simulink model "Tracking_04"  (R2022b)
settings: Solver=ode4  StartTime=0.0  StopTime=50  FixedStep=1e-3  MaxStep=1e-3  RelTol=1e-3
undefined symbols (not defined in the file or in its folder): SF_a, SF_xi2, TT_theta1_init, TT_theta2_init, TT_theta3_init, TT_x_init, TT_y_init, v_sat, w_sat
libraries: simulink x18, dspsigops x3
settings Model: Creator=david  LastModifiedBy=david

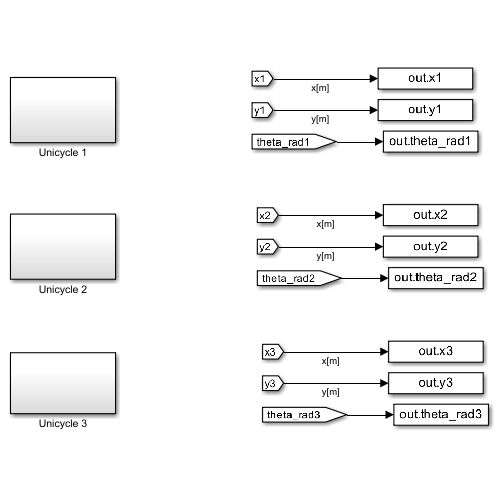
[thumbnail: Simulink's stored preview of the top-level diagram]
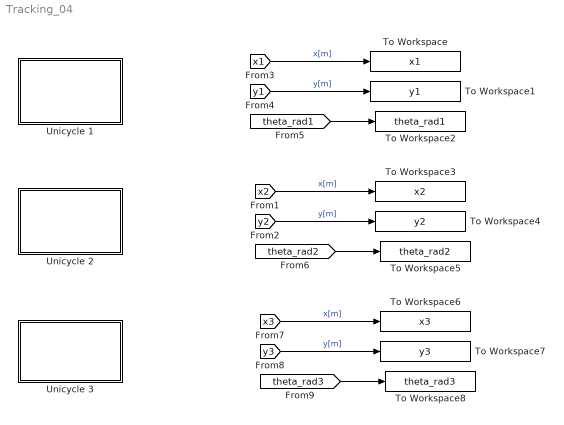
== system Tracking_04 ==
  To Workspace : ToWorkspace  VariableName=x1  SaveFormat=Structure With Time  SampleTime=-1
  To Workspace1 : ToWorkspace  VariableName=y1  SaveFormat=Structure With Time  SampleTime=-1
  To Workspace2 : ToWorkspace  VariableName=theta_rad1  SaveFormat=Structure With Time  SampleTime=-1
  To Workspace3 : ToWorkspace  VariableName=x2  SaveFormat=Structure With Time  SampleTime=-1
  To Workspace4 : ToWorkspace  VariableName=y2  SaveFormat=Structure With Time  SampleTime=-1
  To Workspace5 : ToWorkspace  VariableName=theta_rad2  SaveFormat=Structure With Time  SampleTime=-1
  To Workspace6 : ToWorkspace  VariableName=x3  SaveFormat=Structure With Time  SampleTime=-1
  To Workspace7 : ToWorkspace  VariableName=y3  SaveFormat=Structure With Time  SampleTime=-1
  To Workspace8 : ToWorkspace  VariableName=theta_rad3  SaveFormat=Structure With Time  SampleTime=-1
  Unicycle 1 : Subsystem
  Unicycle 2 : Subsystem
  Unicycle 3 : Subsystem
  wires:
  [x1] -> To Workspace/1  "x[m]"
  [y1] -> To Workspace1/1  "y[m]"
  [theta_rad1] -> To Workspace2/1
  [x2] -> To Workspace3/1  "x[m]"
  [y2] -> To Workspace4/1  "y[m]"
  [theta_rad2] -> To Workspace5/1
  [theta_rad3] -> To Workspace8/1
  [y3] -> To Workspace7/1  "y[m]"
  [x3] -> To Workspace6/1  "x[m]"

== system Tracking_04/Unicycle 1 ==
  State Feedback Approximate Trajectory Controller : Subsystem
  To Workspace : ToWorkspace  VariableName=v1  SaveFormat=Structure With Time  SampleTime=-1
  To Workspace1 : ToWorkspace  VariableName=w1  SaveFormat=Structure With Time  SampleTime=-1
  "Trajectory Generator 1 " : Subsystem
  Unicycle Kinematics : Subsystem
  tag scope: theta_rad1=global, x1=global, y1=global
  wires:
  Unicycle Kinematics/3(theta[rad]) -> [theta_rad1]  "theta[rad]"
  Unicycle Kinematics/2(y[m]) -> [y1]  "y[m]"
  Unicycle Kinematics/1(x[m]) -> [x1]  "x[m]"
  [theta_rad1] -> State Feedback Approximate Trajectory Controller/3(theta[rad])
  [x1] -> State Feedback Approximate Trajectory Controller/1(x[m])
  [y1] -> State Feedback Approximate Trajectory Controller/2(y[m])
  "Trajectory Generator 1 "/1(x_d) -> State Feedback Approximate Trajectory Controller/4(x_d)
  "Trajectory Generator 1 "/2(y_d) -> State Feedback Approximate Trajectory Controller/5(y_d)
  State Feedback Approximate Trajectory Controller/1(v) -> Unicycle Kinematics/1(v[m/s]), To Workspace/1
  State Feedback Approximate Trajectory Controller/2(w) -> Unicycle Kinematics/2(w[rad/s]), To Workspace1/1

== system Tracking_04/Unicycle 2 ==
  State Feedback Approcimate Trajectory Controller : Subsystem
  To Workspace : ToWorkspace  VariableName=v2  SaveFormat=Structure With Time  SampleTime=-1
  To Workspace1 : ToWorkspace  VariableName=w2  SaveFormat=Structure With Time  SampleTime=-1
  "Trajectory Generator 1 " : Subsystem
  Unicycle Kinematics : Subsystem
  tag scope: theta_rad2=global, x2=global, y2=global
  wires:
  Unicycle Kinematics/3(theta[rad]) -> [theta_rad2]  "theta[rad]"
  Unicycle Kinematics/2(y[m]) -> [y2]  "y[m]"
  Unicycle Kinematics/1(x[m]) -> [x2]  "x[m]"
  [theta_rad2] -> State Feedback Approcimate Trajectory Controller/3(theta[rad])
  [x2] -> State Feedback Approcimate Trajectory Controller/1(x[m])
  [y2] -> State Feedback Approcimate Trajectory Controller/2(y[m])
  "Trajectory Generator 1 "/1(x_d) -> State Feedback Approcimate Trajectory Controller/4(x_d)
  "Trajectory Generator 1 "/2(y_d) -> State Feedback Approcimate Trajectory Controller/5(y_d)
  State Feedback Approcimate Trajectory Controller/1(v) -> Unicycle Kinematics/1(v[m/s]), To Workspace/1
  State Feedback Approcimate Trajectory Controller/2(w) -> Unicycle Kinematics/2(w[rad/s]), To Workspace1/1

== system Tracking_04/Unicycle 3 ==
  State Feedback Approximate Trajectory Controller : Subsystem
  To Workspace : ToWorkspace  VariableName=v3  SaveFormat=Structure With Time  SampleTime=-1
  To Workspace1 : ToWorkspace  VariableName=w3  SaveFormat=Structure With Time  SampleTime=-1
  "Trajectory Generator 3 " : Subsystem
  Unicycle Kinematics : Subsystem
  tag scope: theta_rad3=global, x3=global, y3=global
  wires:
  Unicycle Kinematics/3(theta[rad]) -> [theta_rad3]  "theta[rad]"
  Unicycle Kinematics/2(y[m]) -> [y3]  "y[m]"
  Unicycle Kinematics/1(x[m]) -> [x3]  "x[m]"
  [theta_rad3] -> State Feedback Approximate Trajectory Controller/3(theta[rad])
  [x3] -> State Feedback Approximate Trajectory Controller/1(x[m])
  [y3] -> State Feedback Approximate Trajectory Controller/2(y[m])
  "Trajectory Generator 3 "/2(y_d) -> State Feedback Approximate Trajectory Controller/5(y_d)
  "Trajectory Generator 3 "/1(x_d) -> State Feedback Approximate Trajectory Controller/4(x_d)
  State Feedback Approximate Trajectory Controller/1(v) -> Unicycle Kinematics/1(v[m/s]), To Workspace/1
  State Feedback Approximate Trajectory Controller/2(w) -> Unicycle Kinematics/2(w[rad/s]), To Workspace1/1

== system Tracking_04/Unicycle 1/State Feedback Approximate Trajectory Controller ==
  x[m] : Inport
  y[m] : Inport  Port=2
  theta[rad] : Inport  Port=3
  x_d : Inport  Port=4
  y_d : Inport  Port=5
  Controller : Subsystem
  Differential Flatness : Subsystem
  Saturation : Saturate  UpperLimit=v_sat  LowerLimit=-v_sat
  Saturation1 : Saturate  UpperLimit=w_sat  LowerLimit=-w_sat
  v : Outport
  w : Outport  Port=2
  wires:
  Controller/2(w) -> Saturation1/1
  Controller/1(v) -> Saturation/1
  Differential Flatness/3(w_d) -> Controller/3(w_d)
  Differential Flatness/1(q_d) -> Controller/1(q_d)
  Differential Flatness/2(v_d) -> Controller/2(v_d)
  y_d/1 -> Differential Flatness/2(y_d)
  x_d/1 -> Differential Flatness/1(x_d)
  x[m]/1 -> Controller/4(x)
  y[m]/1 -> Controller/5(y)
  theta[rad]/1 -> Controller/6(theta)
  Saturation/1 -> v/1
  Saturation1/1 -> w/1

== system Tracking_04/Unicycle 1/Trajectory Generator 1  ==
  Repeating Sequence : simulink/Sources/Repeating Sequence  rep_seq_t=time  rep_seq_y=y_d1
  Repeating Sequence1 : simulink/Sources/Repeating Sequence  rep_seq_t=time  rep_seq_y=x_d1
  To Workspace2 : ToWorkspace  VariableName=y_d1  SaveFormat=Structure With Time  SampleTime=-1
  To Workspace3 : ToWorkspace  VariableName=x_d1  SaveFormat=Structure With Time  SampleTime=-1
  x_d : Outport
  y_d : Outport  Port=2
  wires:
  Repeating Sequence/1 -> y_d/1, To Workspace2/1
  Repeating Sequence1/1 -> x_d/1, To Workspace3/1

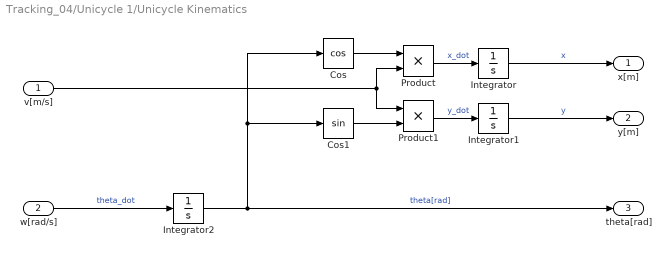
== system Tracking_04/Unicycle 1/Unicycle Kinematics ==
  v[m/s] : Inport
  w[rad/s] : Inport  Port=2
  Cos : Trigonometry  Operator=cos
  Cos1 : Trigonometry
  Integrator : Integrator  InitialCondition=TT_x_init
  Integrator1 : Integrator  InitialCondition=TT_y_init
  Integrator2 : Integrator  InitialCondition=TT_theta1_init
  Product : Product
  Product1 : Product
  x[m] : Outport
  y[m] : Outport  Port=2
  theta[rad] : Outport  Port=3
  wires:
  Integrator/1 -> x[m]/1  "x"
  Integrator1/1 -> y[m]/1  "y"
  w[rad/s]/1 -> Integrator2/1  "theta_dot"
  Integrator2/1 -> Cos/1, Cos1/1, theta[rad]/1  "theta[rad]"
  Product/1 -> Integrator/1  "x_dot"
  Cos1/1 -> Product1/2
  Cos/1 -> Product/1
  v[m/s]/1 -> Product1/1, Product/2
  Product1/1 -> Integrator1/1  "y_dot"

== system Tracking_04/Unicycle 2/State Feedback Approcimate Trajectory Controller ==
  x[m] : Inport
  y[m] : Inport  Port=2
  theta[rad] : Inport  Port=3
  x_d : Inport  Port=4
  y_d : Inport  Port=5
  Controller : Subsystem
  Differential Flatness : Subsystem
  Saturation : Saturate  UpperLimit=v_sat  LowerLimit=-v_sat
  Saturation1 : Saturate  UpperLimit=w_sat  LowerLimit=-w_sat
  v : Outport
  w : Outport  Port=2
  wires:
  Controller/2(w) -> Saturation1/1
  Controller/1(v) -> Saturation/1
  Differential Flatness/3(w_d) -> Controller/3(w_d)
  Differential Flatness/1(q_d) -> Controller/1(q_d)
  Differential Flatness/2(v_d) -> Controller/2(v_d)
  y_d/1 -> Differential Flatness/2(y_d)
  x_d/1 -> Differential Flatness/1(x_d)
  x[m]/1 -> Controller/4(x)
  y[m]/1 -> Controller/5(y)
  theta[rad]/1 -> Controller/6(theta)
  Saturation/1 -> v/1
  Saturation1/1 -> w/1

== system Tracking_04/Unicycle 2/Trajectory Generator 1  ==
  Repeating Sequence : simulink/Sources/Repeating Sequence  rep_seq_t=time  rep_seq_y=y_d2
  Repeating Sequence1 : simulink/Sources/Repeating Sequence  rep_seq_t=time  rep_seq_y=x_d2
  To Workspace2 : ToWorkspace  VariableName=y_d2  SaveFormat=Structure With Time  SampleTime=-1
  To Workspace3 : ToWorkspace  VariableName=x_d2  SaveFormat=Structure With Time  SampleTime=-1
  x_d : Outport
  y_d : Outport  Port=2
  wires:
  Repeating Sequence/1 -> y_d/1, To Workspace2/1
  Repeating Sequence1/1 -> x_d/1, To Workspace3/1

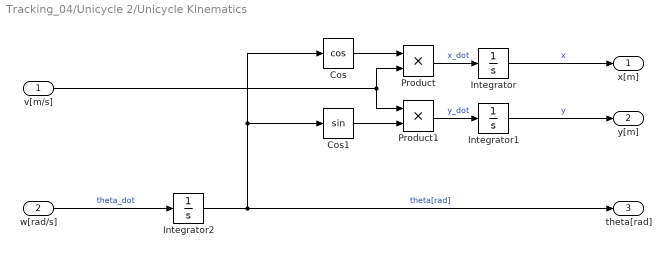
== system Tracking_04/Unicycle 2/Unicycle Kinematics ==
  v[m/s] : Inport
  w[rad/s] : Inport  Port=2
  Cos : Trigonometry  Operator=cos
  Cos1 : Trigonometry
  Integrator : Integrator  InitialCondition=TT_x_init
  Integrator1 : Integrator  InitialCondition=TT_y_init
  Integrator2 : Integrator  InitialCondition=TT_theta2_init
  Product : Product
  Product1 : Product
  x[m] : Outport
  y[m] : Outport  Port=2
  theta[rad] : Outport  Port=3
  wires:
  Integrator/1 -> x[m]/1  "x"
  Integrator1/1 -> y[m]/1  "y"
  w[rad/s]/1 -> Integrator2/1  "theta_dot"
  Integrator2/1 -> Cos/1, Cos1/1, theta[rad]/1  "theta[rad]"
  Product/1 -> Integrator/1  "x_dot"
  Cos1/1 -> Product1/2
  Cos/1 -> Product/1
  v[m/s]/1 -> Product1/1, Product/2
  Product1/1 -> Integrator1/1  "y_dot"

== system Tracking_04/Unicycle 3/State Feedback Approximate Trajectory Controller ==
  x[m] : Inport
  y[m] : Inport  Port=2
  theta[rad] : Inport  Port=3
  x_d : Inport  Port=4
  y_d : Inport  Port=5
  Controller : Subsystem
  Differential Flatness : Subsystem
  Saturation : Saturate  UpperLimit=v_sat  LowerLimit=-v_sat
  Saturation1 : Saturate  UpperLimit=w_sat  LowerLimit=-w_sat
  v : Outport
  w : Outport  Port=2
  wires:
  Controller/2(w) -> Saturation1/1
  Controller/1(v) -> Saturation/1
  Differential Flatness/3(w_d) -> Controller/3(w_d)
  Differential Flatness/1(q_d) -> Controller/1(q_d)
  Differential Flatness/2(v_d) -> Controller/2(v_d)
  y_d/1 -> Differential Flatness/2(y_d)
  x_d/1 -> Differential Flatness/1(x_d)
  x[m]/1 -> Controller/4(x)
  y[m]/1 -> Controller/5(y)
  theta[rad]/1 -> Controller/6(theta)
  Saturation/1 -> v/1
  Saturation1/1 -> w/1

== system Tracking_04/Unicycle 3/Trajectory Generator 3  ==
  Repeating Sequence : simulink/Sources/Repeating Sequence  rep_seq_t=time  rep_seq_y=y_d3
  Repeating Sequence1 : simulink/Sources/Repeating Sequence  rep_seq_t=time  rep_seq_y=x_d3
  To Workspace2 : ToWorkspace  VariableName=y_d3  SaveFormat=Structure With Time  SampleTime=-1
  To Workspace3 : ToWorkspace  VariableName=x_d3  SaveFormat=Structure With Time  SampleTime=-1
  x_d : Outport
  y_d : Outport  Port=2
  wires:
  Repeating Sequence/1 -> y_d/1, To Workspace2/1
  Repeating Sequence1/1 -> x_d/1, To Workspace3/1

== system Tracking_04/Unicycle 3/Unicycle Kinematics ==
  v[m/s] : Inport
  w[rad/s] : Inport  Port=2
  Cos : Trigonometry  Operator=cos
  Cos1 : Trigonometry
  Integrator : Integrator  InitialCondition=TT_x_init
  Integrator1 : Integrator  InitialCondition=TT_y_init
  Integrator2 : Integrator  InitialCondition=TT_theta3_init
  Product : Product
  Product1 : Product
  x[m] : Outport
  y[m] : Outport  Port=2
  theta[rad] : Outport  Port=3
  wires:
  Integrator/1 -> x[m]/1  "x"
  Integrator1/1 -> y[m]/1  "y"
  w[rad/s]/1 -> Integrator2/1  "theta_dot"
  Integrator2/1 -> Cos/1, Cos1/1, theta[rad]/1  "theta[rad]"
  Product/1 -> Integrator/1  "x_dot"
  Cos1/1 -> Product1/2
  Cos/1 -> Product/1
  v[m/s]/1 -> Product1/1, Product/2
  Product1/1 -> Integrator1/1  "y_dot"

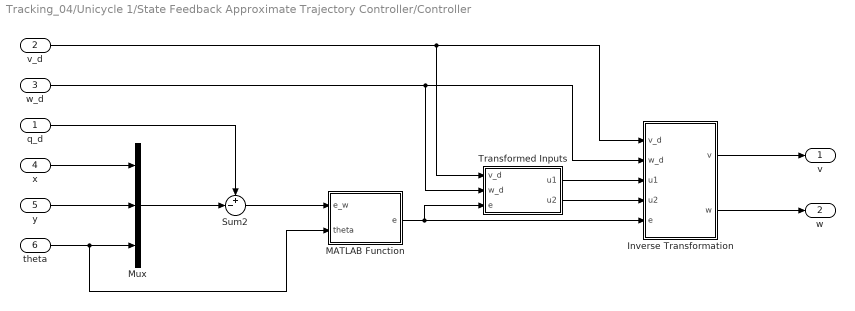
== system Tracking_04/Unicycle 1/State Feedback Approximate Trajectory Controller/Controller ==
  q_d : Inport
  v_d : Inport  Port=2
  w_d : Inport  Port=3
  x : Inport  Port=4
  y : Inport  Port=5
  theta : Inport  Port=6
  Inverse Transformation : MATLAB Function  TreatAsAtomicUnit=on
  MATLAB Function : MATLAB Function  TreatAsAtomicUnit=on
  Mux : Mux  Inputs=3
  Sum2 : Sum  Inputs=+-|
  Transformed Inputs : MATLAB Function  TreatAsAtomicUnit=on
  v : Outport
  w : Outport  Port=2
  wires:
  q_d/1 -> Sum2/1
  MATLAB Function/1(e) -> Inverse Transformation/5(e), Transformed Inputs/3(e)
  Transformed Inputs/1(u1) -> Inverse Transformation/3(u1)
  Transformed Inputs/2(u2) -> Inverse Transformation/4(u2)
  x/1 -> Mux/1
  y/1 -> Mux/2
  theta/1 -> Mux/3, MATLAB Function/2(theta)
  Mux/1 -> Sum2/2
  Sum2/1 -> MATLAB Function/1(e_w)
  w_d/1 -> Inverse Transformation/2(w_d), Transformed Inputs/2(w_d)
  v_d/1 -> Transformed Inputs/1(v_d), Inverse Transformation/1(v_d)
  Inverse Transformation/2(w) -> w/1
  Inverse Transformation/1(v) -> v/1

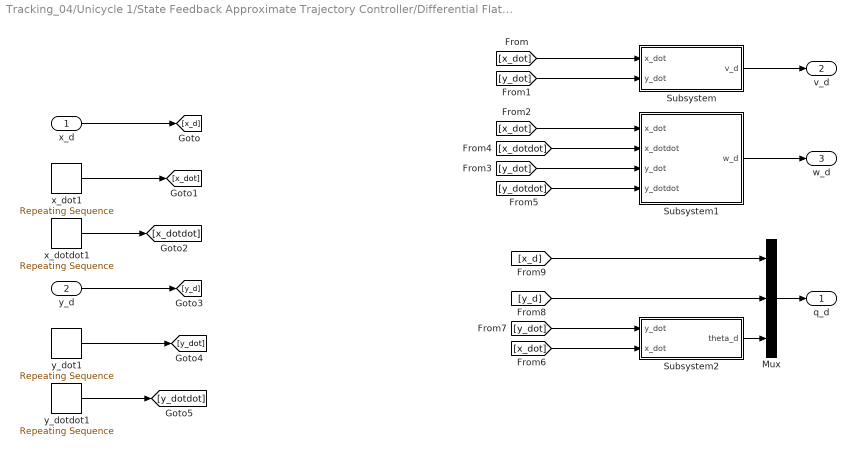
== system Tracking_04/Unicycle 1/State Feedback Approximate Trajectory Controller/Differential Flatness ==
  x_d : Inport
  y_d : Inport  Port=2
  Mux : Mux  Inputs=3
  Subsystem : Subsystem
  Subsystem1 : Subsystem
  Subsystem2 : Subsystem
  x_dot1 : simulink/Sources/Repeating Sequence  rep_seq_t=time  rep_seq_y=x_dot1
  x_dotdot1 : simulink/Sources/Repeating Sequence  rep_seq_t=time  rep_seq_y=x_dotdot1
  y_dot1 : simulink/Sources/Repeating Sequence  rep_seq_t=time  rep_seq_y=y_dot1
  y_dotdot1 : simulink/Sources/Repeating Sequence  rep_seq_t=time  rep_seq_y=y_dotdot1
  q_d : Outport
  v_d : Outport  Port=2
  w_d : Outport  Port=3
  wires:
  Subsystem/1(v_d) -> v_d/1
  [x_dot] -> Subsystem/1(x_dot)
  [y_dot] -> Subsystem/2(y_dot)
  [x_dot] -> Subsystem1/1(x_dot)
  [x_dotdot] -> Subsystem1/2(x_dotdot)
  Subsystem1/1(w_d) -> w_d/1
  [y_dot] -> Subsystem1/3(y_dot)
  [y_dotdot] -> Subsystem1/4(y_dotdot)
  Subsystem2/1(theta_d) -> Mux/3
  [y_d] -> Mux/2
  [x_d] -> Mux/1
  Mux/1 -> q_d/1
  [y_dot] -> Subsystem2/1(y_dot)
  [x_dot] -> Subsystem2/2(x_dot)
  y_dot1/1 -> [y_dot]
  y_dotdot1/1 -> [y_dotdot]
  x_d/1 -> [x_d]
  y_d/1 -> [y_d]
  x_dotdot1/1 -> [x_dotdot]
  x_dot1/1 -> [x_dot]

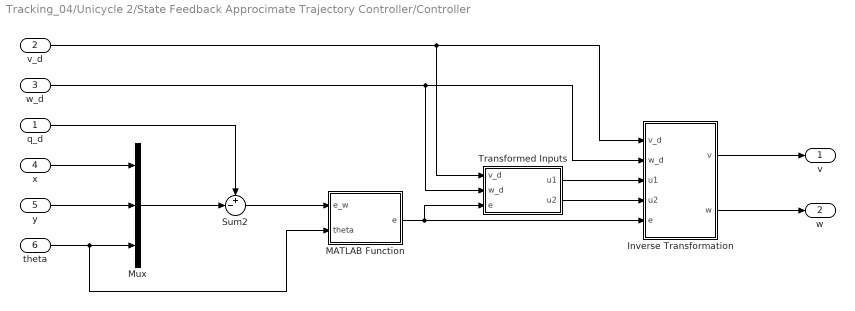
== system Tracking_04/Unicycle 2/State Feedback Approcimate Trajectory Controller/Controller ==
  q_d : Inport
  v_d : Inport  Port=2
  w_d : Inport  Port=3
  x : Inport  Port=4
  y : Inport  Port=5
  theta : Inport  Port=6
  Inverse Transformation : MATLAB Function  TreatAsAtomicUnit=on
  MATLAB Function : MATLAB Function  TreatAsAtomicUnit=on
  Mux : Mux  Inputs=3
  Sum2 : Sum  Inputs=+-|
  Transformed Inputs : MATLAB Function  TreatAsAtomicUnit=on
  v : Outport
  w : Outport  Port=2
  wires:
  q_d/1 -> Sum2/1
  MATLAB Function/1(e) -> Inverse Transformation/5(e), Transformed Inputs/3(e)
  Transformed Inputs/1(u1) -> Inverse Transformation/3(u1)
  Transformed Inputs/2(u2) -> Inverse Transformation/4(u2)
  x/1 -> Mux/1
  y/1 -> Mux/2
  theta/1 -> Mux/3, MATLAB Function/2(theta)
  Mux/1 -> Sum2/2
  Sum2/1 -> MATLAB Function/1(e_w)
  w_d/1 -> Inverse Transformation/2(w_d), Transformed Inputs/2(w_d)
  v_d/1 -> Transformed Inputs/1(v_d), Inverse Transformation/1(v_d)
  Inverse Transformation/2(w) -> w/1
  Inverse Transformation/1(v) -> v/1

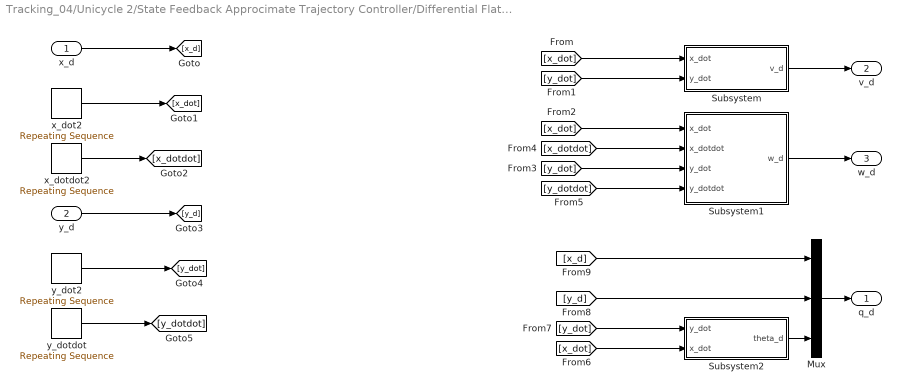
== system Tracking_04/Unicycle 2/State Feedback Approcimate Trajectory Controller/Differential Flatness ==
  x_d : Inport
  y_d : Inport  Port=2
  Mux : Mux  Inputs=3
  Subsystem : Subsystem
  Subsystem1 : Subsystem
  Subsystem2 : Subsystem
  x_dot2 : simulink/Sources/Repeating Sequence  rep_seq_t=time  rep_seq_y=x_dot2
  x_dotdot2 : simulink/Sources/Repeating Sequence  rep_seq_t=time  rep_seq_y=x_dotdot2
  y_dot2 : simulink/Sources/Repeating Sequence  rep_seq_t=time  rep_seq_y=y_dot2
  y_dotdot : simulink/Sources/Repeating Sequence  rep_seq_t=time  rep_seq_y=y_dotdot2
  q_d : Outport
  v_d : Outport  Port=2
  w_d : Outport  Port=3
  wires:
  Subsystem/1(v_d) -> v_d/1
  [x_dot] -> Subsystem/1(x_dot)
  [y_dot] -> Subsystem/2(y_dot)
  [x_dot] -> Subsystem1/1(x_dot)
  [x_dotdot] -> Subsystem1/2(x_dotdot)
  Subsystem1/1(w_d) -> w_d/1
  [y_dot] -> Subsystem1/3(y_dot)
  [y_dotdot] -> Subsystem1/4(y_dotdot)
  Subsystem2/1(theta_d) -> Mux/3
  [y_d] -> Mux/2
  [x_d] -> Mux/1
  Mux/1 -> q_d/1
  [y_dot] -> Subsystem2/1(y_dot)
  [x_dot] -> Subsystem2/2(x_dot)
  y_dot2/1 -> [y_dot]
  y_dotdot/1 -> [y_dotdot]
  x_d/1 -> [x_d]
  y_d/1 -> [y_d]
  x_dotdot2/1 -> [x_dotdot]
  x_dot2/1 -> [x_dot]

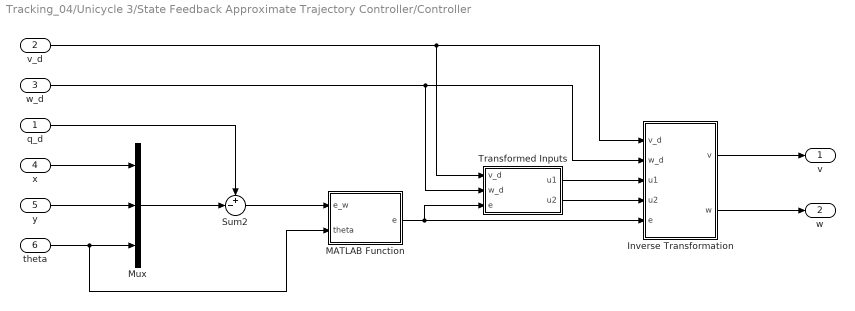
== system Tracking_04/Unicycle 3/State Feedback Approximate Trajectory Controller/Controller ==
  q_d : Inport
  v_d : Inport  Port=2
  w_d : Inport  Port=3
  x : Inport  Port=4
  y : Inport  Port=5
  theta : Inport  Port=6
  Inverse Transformation : MATLAB Function  TreatAsAtomicUnit=on
  MATLAB Function : MATLAB Function  TreatAsAtomicUnit=on
  Mux : Mux  Inputs=3
  Sum2 : Sum  Inputs=+-|
  Transformed Inputs : MATLAB Function  TreatAsAtomicUnit=on
  v : Outport
  w : Outport  Port=2
  wires:
  q_d/1 -> Sum2/1
  MATLAB Function/1(e) -> Transformed Inputs/3(e), Inverse Transformation/5(e)
  Transformed Inputs/1(u1) -> Inverse Transformation/3(u1)
  Transformed Inputs/2(u2) -> Inverse Transformation/4(u2)
  x/1 -> Mux/1
  y/1 -> Mux/2
  theta/1 -> Mux/3, MATLAB Function/2(theta)
  Mux/1 -> Sum2/2
  Sum2/1 -> MATLAB Function/1(e_w)
  w_d/1 -> Inverse Transformation/2(w_d), Transformed Inputs/2(w_d)
  v_d/1 -> Transformed Inputs/1(v_d), Inverse Transformation/1(v_d)
  Inverse Transformation/2(w) -> w/1
  Inverse Transformation/1(v) -> v/1

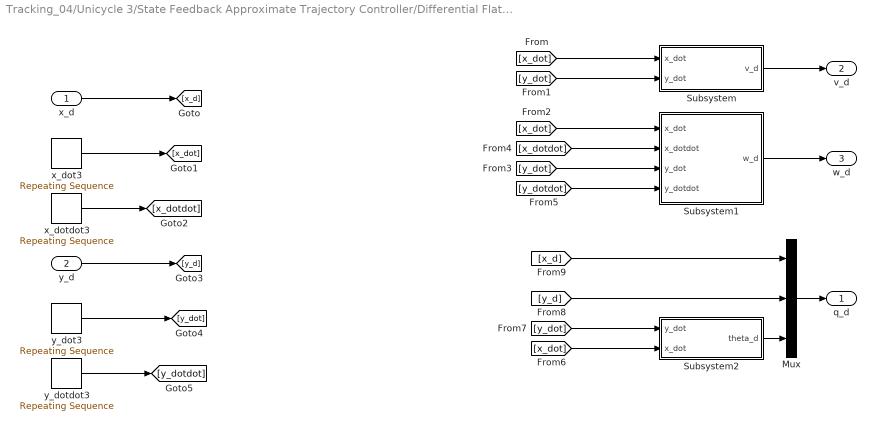
== system Tracking_04/Unicycle 3/State Feedback Approximate Trajectory Controller/Differential Flatness ==
  x_d : Inport
  y_d : Inport  Port=2
  Mux : Mux  Inputs=3
  Subsystem : Subsystem
  Subsystem1 : Subsystem
  Subsystem2 : Subsystem
  x_dot3 : simulink/Sources/Repeating Sequence  rep_seq_t=time  rep_seq_y=x_dot3
  x_dotdot3 : simulink/Sources/Repeating Sequence  rep_seq_t=time  rep_seq_y=x_dotdot3
  y_dot3 : simulink/Sources/Repeating Sequence  rep_seq_t=time  rep_seq_y=y_dot3
  y_dotdot3 : simulink/Sources/Repeating Sequence  rep_seq_t=time  rep_seq_y=y_dotdot3
  q_d : Outport
  v_d : Outport  Port=2
  w_d : Outport  Port=3
  wires:
  x_d/1 -> [x_d]
  Subsystem/1(v_d) -> v_d/1
  x_dotdot3/1 -> [x_dotdot]
  y_d/1 -> [y_d]
  [x_dot] -> Subsystem/1(x_dot)
  [y_dot] -> Subsystem/2(y_dot)
  [x_dot] -> Subsystem1/1(x_dot)
  [x_dotdot] -> Subsystem1/2(x_dotdot)
  Subsystem1/1(w_d) -> w_d/1
  [y_dot] -> Subsystem1/3(y_dot)
  [y_dotdot] -> Subsystem1/4(y_dotdot)
  Subsystem2/1(theta_d) -> Mux/3
  [y_d] -> Mux/2
  [x_d] -> Mux/1
  Mux/1 -> q_d/1
  [y_dot] -> Subsystem2/1(y_dot)
  [x_dot] -> Subsystem2/2(x_dot)
  x_dot3/1 -> [x_dot]
  y_dot3/1 -> [y_dot]
  y_dotdot3/1 -> [y_dotdot]

== system Tracking_04/Unicycle 1/State Feedback Approximate Trajectory Controller/Differential Flatness/Subsystem ==
  x_dot : Inport
  y_dot : Inport  Port=2
  MATLAB Function : MATLAB Function  TreatAsAtomicUnit=on
  Square : Math  Operator=square
  Square Root : Sqrt
  Square1 : Math  Operator=square
  Sum : Sum
  v_d : Outport
  wires:
  x_dot/1 -> Square/1
  y_dot/1 -> Square1/1
  Square/1 -> Sum/1
  Square1/1 -> Sum/2
  Square Root/1 -> MATLAB Function/1("u ")
  Sum/1 -> Square Root/1
  MATLAB Function/1(u) -> v_d/1

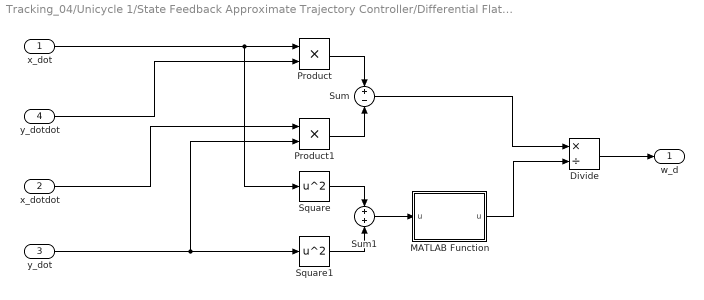
== system Tracking_04/Unicycle 1/State Feedback Approximate Trajectory Controller/Differential Flatness/Subsystem1 ==
  x_dot : Inport
  x_dotdot : Inport  Port=2
  y_dot : Inport  Port=3
  y_dotdot : Inport  Port=4
  Divide : Product  Inputs=*/
  MATLAB Function : MATLAB Function  TreatAsAtomicUnit=on
  Product : Product
  Product1 : Product
  Square : Math  Operator=square
  Square1 : Math  Operator=square
  Sum : Sum  Inputs=+-
  Sum1 : Sum
  w_d : Outport
  wires:
  Product/1 -> Sum/1
  Product1/1 -> Sum/2
  Sum/1 -> Divide/1
  Divide/1 -> w_d/1
  x_dot/1 -> Square/1, Product/1
  y_dotdot/1 -> Product/2
  y_dot/1 -> Product1/2, Square1/1
  MATLAB Function/1(u) -> Divide/2
  Sum1/1 -> MATLAB Function/1("u ")
  Square/1 -> Sum1/1
  Square1/1 -> Sum1/2
  x_dotdot/1 -> Product1/1

== system Tracking_04/Unicycle 1/State Feedback Approximate Trajectory Controller/Differential Flatness/Subsystem2 ==
  y_dot : Inport
  x_dot : Inport  Port=2
  Atan2 : Trigonometry  Operator=atan2
  Unwrap : dspsigops/Unwrap  tol=pi  InputProcessing=Columns as channels (frame based)  running=off
  theta_d : Outport
  wires:
  y_dot/1 -> Atan2/1
  x_dot/1 -> Atan2/2
  Atan2/1 -> Unwrap/1
  Unwrap/1 -> theta_d/1

== system Tracking_04/Unicycle 2/State Feedback Approcimate Trajectory Controller/Differential Flatness/Subsystem ==
  x_dot : Inport
  y_dot : Inport  Port=2
  MATLAB Function : MATLAB Function  TreatAsAtomicUnit=on
  Square : Math  Operator=square
  Square Root : Sqrt
  Square1 : Math  Operator=square
  Sum : Sum
  v_d : Outport
  wires:
  x_dot/1 -> Square/1
  y_dot/1 -> Square1/1
  Square/1 -> Sum/1
  Square1/1 -> Sum/2
  Square Root/1 -> MATLAB Function/1("u ")
  Sum/1 -> Square Root/1
  MATLAB Function/1(u) -> v_d/1

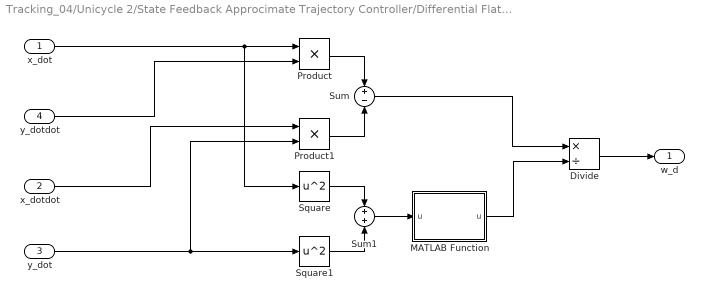
== system Tracking_04/Unicycle 2/State Feedback Approcimate Trajectory Controller/Differential Flatness/Subsystem1 ==
  x_dot : Inport
  x_dotdot : Inport  Port=2
  y_dot : Inport  Port=3
  y_dotdot : Inport  Port=4
  Divide : Product  Inputs=*/
  MATLAB Function : MATLAB Function  TreatAsAtomicUnit=on
  Product : Product
  Product1 : Product
  Square : Math  Operator=square
  Square1 : Math  Operator=square
  Sum : Sum  Inputs=+-
  Sum1 : Sum
  w_d : Outport
  wires:
  Product/1 -> Sum/1
  Product1/1 -> Sum/2
  Sum/1 -> Divide/1
  Divide/1 -> w_d/1
  x_dot/1 -> Square/1, Product/1
  y_dotdot/1 -> Product/2
  y_dot/1 -> Product1/2, Square1/1
  MATLAB Function/1(u) -> Divide/2
  Sum1/1 -> MATLAB Function/1("u ")
  Square/1 -> Sum1/1
  Square1/1 -> Sum1/2
  x_dotdot/1 -> Product1/1

== system Tracking_04/Unicycle 2/State Feedback Approcimate Trajectory Controller/Differential Flatness/Subsystem2 ==
  y_dot : Inport
  x_dot : Inport  Port=2
  Atan2 : Trigonometry  Operator=atan2
  Unwrap : dspsigops/Unwrap  tol=pi  InputProcessing=Columns as channels (frame based)  running=off
  theta_d : Outport
  wires:
  y_dot/1 -> Atan2/1
  x_dot/1 -> Atan2/2
  Atan2/1 -> Unwrap/1
  Unwrap/1 -> theta_d/1

== system Tracking_04/Unicycle 3/State Feedback Approximate Trajectory Controller/Differential Flatness/Subsystem ==
  x_dot : Inport
  y_dot : Inport  Port=2
  MATLAB Function : MATLAB Function  TreatAsAtomicUnit=on
  Square : Math  Operator=square
  Square Root : Sqrt
  Square1 : Math  Operator=square
  Sum : Sum
  v_d : Outport
  wires:
  x_dot/1 -> Square/1
  y_dot/1 -> Square1/1
  Square/1 -> Sum/1
  Square1/1 -> Sum/2
  Square Root/1 -> MATLAB Function/1("u ")
  Sum/1 -> Square Root/1
  MATLAB Function/1(u) -> v_d/1

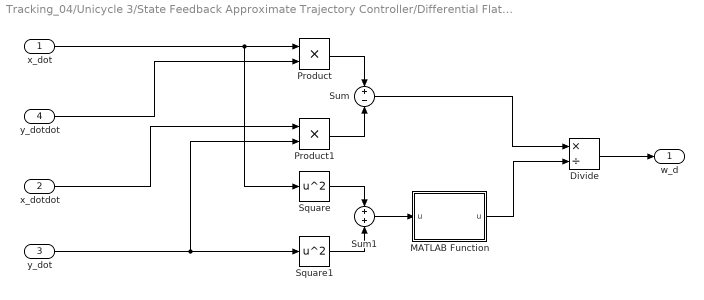
== system Tracking_04/Unicycle 3/State Feedback Approximate Trajectory Controller/Differential Flatness/Subsystem1 ==
  x_dot : Inport
  x_dotdot : Inport  Port=2
  y_dot : Inport  Port=3
  y_dotdot : Inport  Port=4
  Divide : Product  Inputs=*/
  MATLAB Function : MATLAB Function  TreatAsAtomicUnit=on
  Product : Product
  Product1 : Product
  Square : Math  Operator=square
  Square1 : Math  Operator=square
  Sum : Sum  Inputs=+-
  Sum1 : Sum
  w_d : Outport
  wires:
  Product/1 -> Sum/1
  Product1/1 -> Sum/2
  Sum/1 -> Divide/1
  Divide/1 -> w_d/1
  x_dot/1 -> Square/1, Product/1
  y_dotdot/1 -> Product/2
  y_dot/1 -> Product1/2, Square1/1
  Sum1/1 -> MATLAB Function/1("u ")
  Square/1 -> Sum1/1
  Square1/1 -> Sum1/2
  x_dotdot/1 -> Product1/1
  MATLAB Function/1(u) -> Divide/2

== system Tracking_04/Unicycle 3/State Feedback Approximate Trajectory Controller/Differential Flatness/Subsystem2 ==
  y_dot : Inport
  x_dot : Inport  Port=2
  Atan2 : Trigonometry  Operator=atan2
  Unwrap : dspsigops/Unwrap  tol=pi  InputProcessing=Columns as channels (frame based)  running=off
  theta_d : Outport
  wires:
  y_dot/1 -> Atan2/1
  x_dot/1 -> Atan2/2
  Atan2/1 -> Unwrap/1
  Unwrap/1 -> theta_d/1

== matlab function Tracking_04/Unicycle 2/State Feedback Approcimate Trajectory Controller/Controller/Inverse Transformation ==
  data: v_d input; w_d input; u1 input; v output size=1; u2 input; w output size=1; e input
function [v, w] = fcn(v_d, w_d, u1, u2, e)

v = v_d*cos(e(3))-u1;
w=w_d-u2;

== matlab function Tracking_04/Unicycle 2/State Feedback Approcimate Trajectory Controller/Controller/MATLAB Function ==
  data: e_w input; e output; theta input
function e  = fcn(e_w, theta)

R=[cos(theta) sin(theta) 0; -sin(theta) cos(theta) 0; 0 0 1];

e=R*e_w;

if(abs(e(3))>=2*pi-1e-4)
    e(3) = 0;
end

== matlab function Tracking_04/Unicycle 2/State Feedback Approcimate Trajectory Controller/Controller/Transformed Inputs ==
  data: SF_a parameter; SF_xi2 parameter; v_d input; w_d input; e input; u1 output; u2 output
function [u1, u2] = fcn(SF_a, SF_xi2, v_d, w_d, e)

% calculatring values of K
k_1=2*SF_xi2*SF_a;
k_2=(SF_a^2-w_d^2)/(v_d);
k_3=k_1;

% calculating values of u
u1=-k_1*e(1);
u2=-k_2*e(2)-k_3*e(3);

== matlab function Tracking_04/Unicycle 3/State Feedback Approximate Trajectory Controller/Differential Flatness/Subsystem/MATLAB Function ==
  data: u input; u output
function u = fcn(u)

if abs(u)<1e-4
    if u>=0
        u=1e-4;
    else
        u=-1e-4;
    end
else
    u=u;
end

== matlab function Tracking_04/Unicycle 2/State Feedback Approcimate Trajectory Controller/Differential Flatness/Subsystem/MATLAB Function ==
  data: u input; u output
function u = fcn(u)

if abs(u)<1e-4
    if u>=0
        u=1e-4;
    else
        u=-1e-4;
    end
else
    u=u;
end

== matlab function Tracking_04/Unicycle 3/State Feedback Approximate Trajectory Controller/Differential Flatness/Subsystem1/MATLAB Function ==
  data: u input; u output
function u = fcn(u)

if abs(u)<1e-4
    if u>=0
        u=1e-4;
    else
        u=-1e-4;
    end
else
    u=u;
end

== matlab function Tracking_04/Unicycle 2/State Feedback Approcimate Trajectory Controller/Differential Flatness/Subsystem1/MATLAB Function ==
  data: u input; u output
function u = fcn(u)

if abs(u)<1e-4
    if u>=0
        u=1e-4;
    else
        u=-1e-4;
    end
else
    u=u;
end

== matlab function Tracking_04/Unicycle 1/State Feedback Approximate Trajectory Controller/Differential Flatness/Subsystem/MATLAB Function ==
  data: u input; u output
function u = fcn(u)

if abs(u)<1e-4
    if u>=0
        u=1e-4;
    else
        u=-1e-4;
    end
else
    u=u;
end

== matlab function Tracking_04/Unicycle 3/State Feedback Approximate Trajectory Controller/Controller/Inverse Transformation ==
  data: v_d input; w_d input; u1 input; v output size=1; u2 input; w output size=1; e input
function [v, w] = fcn(v_d, w_d, u1, u2, e)

v = v_d*cos(e(3))-u1;
w = w_d-u2;

== matlab function Tracking_04/Unicycle 1/State Feedback Approximate Trajectory Controller/Controller/Inverse Transformation ==
  data: v_d input; w_d input; u1 input; v output size=1; u2 input; w output size=1; e input
function [v, w] = fcn(v_d, w_d, u1, u2, e)

v = v_d*cos(e(3))-u1;
w=w_d-u2;

== matlab function Tracking_04/Unicycle 1/State Feedback Approximate Trajectory Controller/Controller/MATLAB Function ==
  data: e_w input; e output; theta input
function e  = fcn(e_w, theta)

R=[cos(theta) sin(theta) 0; -sin(theta) cos(theta) 0; 0 0 1];

e=R*e_w;

if(abs(e(3))>=2*pi-1e-4)
    e(3) = 0;
end

== matlab function Tracking_04/Unicycle 1/State Feedback Approximate Trajectory Controller/Controller/Transformed Inputs ==
  data: SF_a parameter; SF_xi2 parameter; v_d input; w_d input; e input; u1 output; u2 output
function [u1, u2] = fcn(SF_a, SF_xi2, v_d, w_d, e)

% calculatring values of K
k_1=2*SF_xi2*SF_a;
k_2=(SF_a^2-w_d^2)/(v_d);
k_3=k_1;

% calculating values of u
u1=-k_1*e(1);
u2=-k_2*e(2)-k_3*e(3);

== matlab function Tracking_04/Unicycle 1/State Feedback Approximate Trajectory Controller/Differential Flatness/Subsystem1/MATLAB Function ==
  data: u input; u output
function u = fcn(u)

if abs(u)<1e-4
    if u>=0
        u=1e-4;
    else
        u=-1e-4;
    end
else
    u=u;
end

== matlab function Tracking_04/Unicycle 3/State Feedback Approximate Trajectory Controller/Controller/MATLAB Function ==
  data: e_w input; e output; theta input
function e  = fcn(e_w, theta)

R=[cos(theta) sin(theta) 0; -sin(theta) cos(theta) 0; 0 0 1];

e=R*e_w;
if(abs(e(3))>=2*pi-1e-4)
    e(3) = 0;
end

== matlab function Tracking_04/Unicycle 3/State Feedback Approximate Trajectory Controller/Controller/Transformed Inputs ==
  data: SF_a parameter; SF_xi2 parameter; v_d input; w_d input; e input; u1 output; u2 output
function [u1, u2] = fcn(SF_a, SF_xi2, v_d, w_d, e)

% calculatring values of K
k_1=2*SF_xi2*SF_a;
k_2=(SF_a^2-w_d^2)/(v_d);
k_3=k_1;

% calculating values of u
u1=-k_1*e(1);
u2=-k_2*e(2)-k_3*e(3);
